simulink library "ADV_IP_MASTER"  (Simulink 8.6)
settings: Solver=VariableStepAuto  StartTime=0.0  StopTime=10.0  RelTol=1e-3
libraries: cdsEpicsOut x45, cdsFiltCtrl x25, cdsFilt x19, cdsEpicsIn x16, cdsTP x6, cdsMuxMatrix x4, VIS_LIB x1, cdsRampMuxMatrix x1, cdsFunctionCall x1, SIXOSEM_F_WD_AC_MASTER x1, SIXOSEM_F_STAGE_MASTER x1
(part 1 of 5)
settings Model: Creator=controls  LastModifiedBy=controls

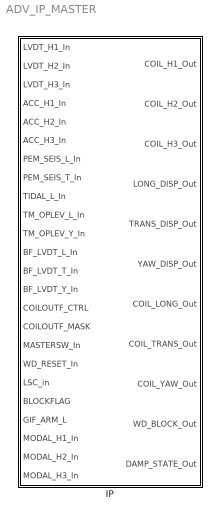
== system ADV_IP_MASTER ==
  IP : Subsystem

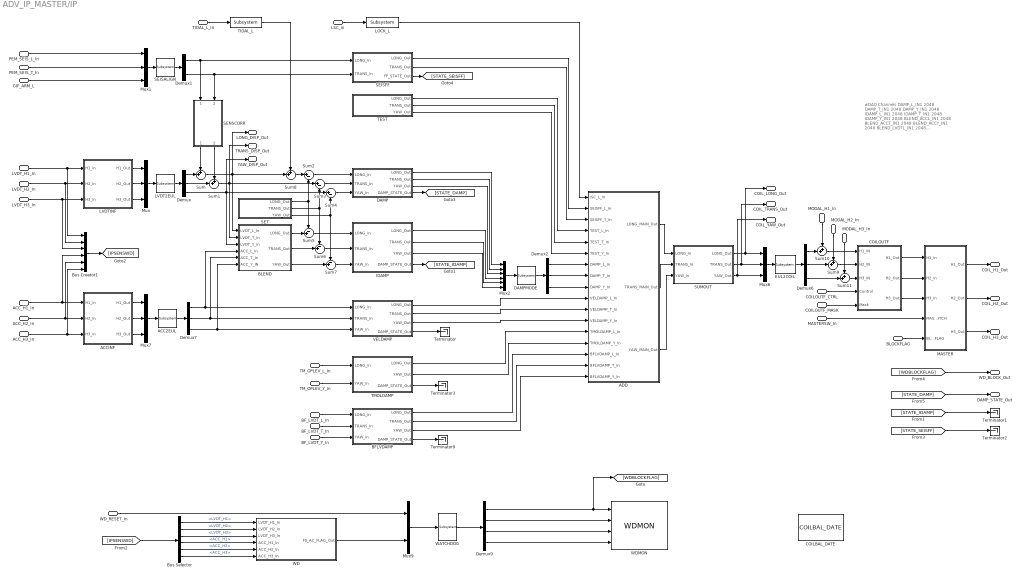
== system ADV_IP_MASTER/IP ==
  note: #DAQ Channels
      | DAMP_L_IN1 2048
      | DAMP_T_IN1 2048
      | DAMP_Y_IN1 2048
      | IDAMP_L_IN1 2048
      | IDAMP_T_IN1 2048
      | IDAMP_Y_IN1 2048
      | BLEND_ACCL_IN1 2048
      | BLEND_ACCT_IN1 2048
      | BLEND_ACCY_IN1 2048
      | BLEND_LVDTL_IN1 2048
      | BLEND_LVDTT_IN1 2048
      | BLEND_LVDTY_IN1 2048
      | DAMP_L_OUT 256
      | DAMP_T_OUT 256
      | DAMP_Y_OUT 256
      | IDAMP_L_OUT 256
      | IDAMP_T_OUT 256
      | IDAMP_Y_OUT 256
      | SEISFF_L_OUT 256
      | SEISFF_T_OUT 256
      | LOCK_L_OUT 256
      | TIDAL_L_OUT 32
  LVDT_H1_In : Inport
  LVDT_H2_In : Inport  Port=2
  LVDT_H3_In : Inport  Port=3
  ACC_H1_In : Inport  Port=4
  ACC_H2_In : Inport  Port=5
  ACC_H3_In : Inport  Port=6
  PEM_SEIS_L_In : Inport  Port=7
  PEM_SEIS_T_In : Inport  Port=8
  TIDAL_L_In : Inport  Port=9
  TM_OPLEV_L_In : Inport  Port=10
  TM_OPLEV_Y_In : Inport  Port=11
  BF_LVDT_L_In : Inport  Port=12
  BF_LVDT_T_In : Inport  Port=13
  BF_LVDT_Y_In : Inport  Port=14
  COILOUTF_CTRL : Inport  Port=15
  COILOUTF_MASK : Inport  Port=16
  MASTERSW_In : Inport  Port=17
  WD_RESET_In : Inport  Port=18
  LSC_in : Inport  Port=19
  BLOCKFLAG : Inport  Port=20
  GIF_ARM_L : Inport  Port=21
  MODAL_H1_In : Inport  Port=22
  MODAL_H2_In : Inport  Port=23
  MODAL_H3_In : Inport  Port=24
  ACC2EUL : cdsMuxMatrix/Subsystem  Tag=cdsMuxMatrix  Description=|
      | ADL=SUS_INMATRIX.adl
      | SCRIPT=generate_KisselButton.py 4 5 #CHANNEL# > #TARGET_DIR#/#FULL_PART_NAME#_KB.adl
      settings: AttributesFormatString=%<Tag>
  ACCINF : Subsystem
  ADD : Subsystem
  BFLVDAMP : Subsystem
  BLEND : Subsystem
  Bus Creator1 : BusCreator  Inputs='LVDT_H1','LVDT_H2','LVDT_H3','ACC_H1','ACC_H2','ACC_H3'
  Bus Selector : BusSelector  OutputSignals=LVDT_H1,LVDT_H2,LVDT_H3,ACC_H1,ACC_H2,ACC_H3
  COILBAL_DATE : VIS_LIB/COILBAL_DATE
  COILOUTF : Subsystem
  DAMP : Subsystem
  DAMPMODE : cdsRampMuxMatrix/Subsystem  Tag=cdsRampMuxMatrix
      settings: AttributesFormatString=%<Tag>
  Demux{,2,6..7} (4 alike) : Demux  Outputs=3
  Demux1 : Demux  Outputs=2
  Demux9 : Demux
  EUL2COIL : cdsMuxMatrix/Subsystem  Tag=cdsMuxMatrix  Description=|
      | ADL=SUS_INMATRIX.adl
      | SCRIPT=generate_KisselButton.py 4 5 #CHANNEL# > #TARGET_DIR#/#FULL_PART_NAME#_KB.adl
      settings: AttributesFormatString=%<Tag>
  IDAMP : Subsystem
  LOCK_L : cdsFilt/Subsystem  Tag=cdsFilt  Description=|
      | Purpose:                                                                                                                                                                                                                                  
      | Standard CDS IIR filter module.                                                                                                                                                                                                           
      |                                                                                                                                                                                                                                           
      | Operation:                                                                                                                                                                                                                                
      | Consists of 10 second order section IIR filters, plus a ramped gain stage. In FE code, also provides pre-defined test points and excitation channel inputs. The filter coefficients are defined in the LIGO system using the 'foton' tool.
      |                                                                                                                                                                                                                                           
      | Usage:                                                                                                                                                                                                                                    
      | Name the part with the desired filter module name.
      settings: AttributesFormatString=%<Tag>
  LVDT2EUL : cdsMuxMatrix/Subsystem  Tag=cdsMuxMatrix  Description=|
      | ADL=SUS_INMATRIX.adl
      | SCRIPT=generate_KisselButton.py 4 5 #CHANNEL# > #TARGET_DIR#/#FULL_PART_NAME#_KB.adl
      settings: AttributesFormatString=%<Tag>
  LVDTINF : Subsystem
  MASTER : Subsystem
  Mux{,1,6..7} (4 alike) : Mux  Inputs=3
  Mux2 : Mux  Inputs=6
  Mux9 : Mux  Inputs=2
  SEISALIGN : cdsMuxMatrix/Subsystem  Tag=cdsMuxMatrix  Description=|
      | ADL=SUS_INMATRIX.adl
      | SCRIPT=generate_KisselButton.py 4 5 #CHANNEL# > #TARGET_DIR#/#FULL_PART_NAME#_KB.adl
      settings: AttributesFormatString=%<Tag>
  SEISFF : Subsystem
  SENSCORR : Subsystem
  SET : Subsystem
  SUMOUT : Subsystem
  Sum{,1,8..11} (6 alike) : Sum  Inputs=++|
  Sum2 : Sum  Inputs=|+-
  Sum3 : Sum  Inputs=|+-
  Sum4 : Sum  Inputs=|+-
  Sum5 : Sum  Inputs=-+|
  Sum6 : Sum  Inputs=-+|
  Sum7 : Sum  Inputs=-+|
  TEST : Subsystem
  TIDAL_L : cdsFilt/Subsystem  Tag=cdsFilt  Description=|
      | Purpose:                                                                                                                                                                                                                                  
      | Standard CDS IIR filter module.                                                                                                                                                                                                           
      |                                                                                                                                                                                                                                           
      | Operation:                                                                                                                                                                                                                                
      | Consists of 10 second order section IIR filters, plus a ramped gain stage. In FE code, also provides pre-defined test points and excitation channel inputs. The filter coefficients are defined in the LIGO system using the 'foton' tool.
      |                                                                                                                                                                                                                                           
      | Usage:                                                                                                                                                                                                                                    
      | Name the part with the desired filter module name.
      settings: AttributesFormatString=%<Tag>
  TMOLDAMP : Subsystem
  Terminator{,1..3,9} (5 alike) : Terminator
  VELDAMP : Subsystem
  WATCHDOG : cdsFunctionCall/Subsystem  Tag=cdsFunctionCall  Description=inline OSEMWATCHDOG /opt/rtcds/userapps/release/vis/common/src/WATCHDOG.c
      settings: AttributesFormatString=%<Tag>\n%<Description>
  WD : Subsystem
  WDMON : SIXOSEM_F_STAGE_MASTER/SIXOSEM_F_STAGE_MASTER/WDMON
  COIL_H1_Out : Outport
  COIL_H2_Out : Outport  Port=2
  COIL_H3_Out : Outport  Port=3
  LONG_DISP_Out : Outport  Port=4
  TRANS_DISP_Out : Outport  Port=5
  YAW_DISP_Out : Outport  Port=6
  COIL_LONG_Out : Outport  Port=7
  COIL_TRANS_Out : Outport  Port=8
  COIL_YAW_Out : Outport  Port=9
  WD_BLOCK_Out : Outport  Port=10
  DAMP_STATE_Out : Outport  Port=11
  wires:
  MODAL_H3_In/1 -> Sum11/1
  MODAL_H2_In/1 -> Sum9/1
  Demux6/3 -> Sum11/2
  Sum11/1 -> COILOUTF/3(H3_IN)
  Sum9/1 -> COILOUTF/2(H2_IN)
  Demux6/2 -> Sum9/2
  Sum10/1 -> COILOUTF/1(H1_IN)
  Demux6/1 -> Sum10/2
  MODAL_H1_In/1 -> Sum10/1
  [STATE_DAMP] -> DAMP_STATE_Out/1
  [WDBLOCKFLAG] -> WD_BLOCK_Out/1
  COILOUTF_MASK/1 -> COILOUTF/5(Mask)
  COILOUTF_CTRL/1 -> COILOUTF/4(Control)
  TEST/3(YAW_Out) -> ADD/6(TEST_Y_In)
  TEST/2(TRANS_Out) -> ADD/5(TEST_T_In)
  TEST/1(LONG_Out) -> ADD/4(TEST_L_In)
  BLEND/3(YAW_Out) -> Sum7/2
  BLEND/2(TRANS_Out) -> Sum6/2
  BLOCKFLAG/1 -> MASTER/5(BLOCKFLAG)
  Bus Creator1/1 -> [IPSENSWD]
  ACC_H3_In/1 -> ACCINF/3(H3_In), Bus Creator1/6
  ACC_H2_In/1 -> ACCINF/2(H2_In), Bus Creator1/5
  ACC_H1_In/1 -> ACCINF/1(H1_In), Bus Creator1/4
  LVDT_H3_In/1 -> LVDTINF/3(H3_In), Bus Creator1/3
  LVDT_H2_In/1 -> LVDTINF/2(H2_In), Bus Creator1/2
  LVDT_H1_In/1 -> LVDTINF/1(H1_In), Bus Creator1/1
  WATCHDOG/1 -> Demux9/1
  Mux9/1 -> WATCHDOG/1
  Demux9/4 -> WDMON/4
  Demux9/3 -> WDMON/3
  Demux9/2 -> WDMON/2
  Demux9/1 -> WDMON/1, [WDBLOCKFLAG]
  Bus Selector/5 -> WD/5(ACC_H2_In)  "<ACC_H2>"
  Bus Selector/6 -> WD/6(ACC_H3_In)  "<ACC_H3>"
  Bus Selector/4 -> WD/4(ACC_H1_In)  "<ACC_H1>"
  Bus Selector/3 -> WD/3(LVDT_H3_In)  "<LVDT_H3>"
  Bus Selector/2 -> WD/2(LVDT_H2_In)  "<LVDT_H2>"
  Bus Selector/1 -> WD/1(LVDT_H1_In)  "<LVDT_H1>"
  [IPSENSWD] -> Bus Selector/1
  WD/1(F0_AC_FLAG_Out) -> Mux9/2
  WD_RESET_In/1 -> Mux9/1
  MASTERSW_In/1 -> MASTER/4(MASTERSWITCH)
  COILOUTF/3(H3_Out) -> MASTER/3(H3_In)
  COILOUTF/2(H2_Out) -> MASTER/2(H2_In)
  COILOUTF/1(H1_Out) -> MASTER/1(H1_In)
  MASTER/3(H3_Out) -> COIL_H3_Out/1
  MASTER/2(H2_Out) -> COIL_H2_Out/1
  MASTER/1(H1_Out) -> COIL_H1_Out/1
  EUL2COIL/1 -> Demux6/1
  Mux6/1 -> EUL2COIL/1
  Demux7/3 -> BLEND/6(ACC_Y_IN), VELDAMP/3(YAW_In)
  Demux7/2 -> BLEND/5(ACC_T_In), VELDAMP/2(TRANS_In)
  Demux7/1 -> BLEND/4(ACC_L_In), VELDAMP/1(LONG_In)
  Demux/3 -> Sum4/1, BLEND/3(LVDT_Y_In), YAW_DISP_Out/1
  Sum1/1 -> Sum3/1, BLEND/2(LVDT_T_In), TRANS_DISP_Out/1
  Sum/1 -> Sum8/2, LONG_DISP_Out/1, BLEND/1(LVDT_L_In)
  ACC2EUL/1 -> Demux7/1
  ACCINF/2(H2_Out) -> Mux7/2
  ACCINF/3(H3_Out) -> Mux7/3
  ACCINF/1(H1_Out) -> Mux7/1
  Mux7/1 -> ACC2EUL/1
  LVDT2EUL/1 -> Demux/1
  Mux/1 -> LVDT2EUL/1
  LVDTINF/3(H3_Out) -> Mux/3
  LVDTINF/2(H2_Out) -> Mux/2
  LVDTINF/1(H1_Out) -> Mux/1
  VELDAMP/1(LONG_Out) -> ADD/10(VELDAMP_L_In)
  VELDAMP/2(TRANS_Out) -> ADD/11(VELDAMP_T_In)
  VELDAMP/3(YAW_Out) -> ADD/12(VELDAMP_Y_In)
  VELDAMP/4(DAMP_STATE_Out) -> Terminator/1
  LSC_in/1 -> LOCK_L/1
  BLEND/1(LONG_Out) -> Sum5/2
  DAMP/4(DAMP_STATE_Out) -> [STATE_DAMP]
  IDAMP/4(DAMP_STATE_Out) -> [STATE_IDAMP]
  [STATE_IDAMP] -> Terminator1/1
  Demux/1 -> Sum/2
  SENSCORR/1(SC_L_Out) -> Sum/1
  Demux/2 -> Sum1/2
  SENSCORR/2(SC_T_Out) -> Sum1/1
  SEISFF/3(FF_STATE_Out) -> [STATE_SEISFF]
  SEISFF/2(TRANS_Out) -> ADD/3(SEISFF_T_In)
  SEISFF/1(LONG_Out) -> ADD/2(SEISFF_L_In)
  [STATE_SEISFF] -> Terminator2/1
  SUMOUT/3(YAW_Out) -> COIL_YAW_Out/1, Mux6/3
  SUMOUT/1(LONG_Out) -> COIL_LONG_Out/1, Mux6/1
  SUMOUT/2(TRANS_Out) -> COIL_TRANS_Out/1, Mux6/2
  ADD/2(TRANS_MAIN_Out) -> SUMOUT/2(TRANS_In)
  ADD/1(LONG_MAIN_Out) -> SUMOUT/1(LONG_In)
  ADD/3(YAW_MAIN_Out) -> SUMOUT/3(YAW_In)
  PEM_SEIS_T_In/1 -> Mux1/2
  PEM_SEIS_L_In/1 -> Mux1/1
  Mux1/1 -> SEISALIGN/1
  SEISALIGN/1 -> Demux1/1
  Demux1/2 -> SENSCORR/2(SEIS_T_In), SEISFF/2(TRANS_In)
  Demux1/1 -> SENSCORR/1(SEIS_L_In), SEISFF/1(LONG_In)
  Sum2/1 -> DAMP/1(LONG_In)
  Sum3/1 -> DAMP/2(TRANS_In)
  Sum4/1 -> DAMP/3(YAW_In)
  SET/1(LONG_Out) -> Sum5/1, Sum2/2
  SET/2(TRANS_Out) -> Sum3/2, Sum6/1
  SET/3(YAW_Out) -> Sum7/1, Sum4/2
  Sum7/1 -> IDAMP/3(YAW_In)
  Sum6/1 -> IDAMP/2(TRANS_In)
  Sum5/1 -> IDAMP/1(LONG_In)
  Mux2/1 -> DAMPMODE/1
  DAMPMODE/1 -> Demux2/1
  DAMP/3(YAW_Out) -> Mux2/3
  DAMP/2(TRANS_Out) -> Mux2/2
  DAMP/1(LONG_Out) -> Mux2/1
  IDAMP/3(YAW_Out) -> Mux2/6
  IDAMP/2(TRANS_Out) -> Mux2/5
  IDAMP/1(LONG_Out) -> Mux2/4
  Demux2/1 -> ADD/7(DAMP_L_In)
  Demux2/2 -> ADD/8(DAMP_T_In)
  Demux2/3 -> ADD/9(DAMP_Y_In)
  LOCK_L/1 -> ADD/1(ISC_L_In)
  TMOLDAMP/3(DAMP_STATE_Out) -> Terminator3/1
  TM_OPLEV_L_In/1 -> TMOLDAMP/1(LONG_In)
  TM_OPLEV_Y_In/1 -> TMOLDAMP/2(YAW_In)
  BFLVDAMP/4(DAMP_STATE_Out) -> Terminator9/1
  TMOLDAMP/1(LONG_Out) -> ADD/13(TMOLDAMP_L_In)
  TMOLDAMP/2(YAW_Out) -> ADD/14(TMOLDAMP_Y_In)
  BFLVDAMP/3(YAW_Out) -> ADD/17(BFLVDAMP_Y_In)
  BFLVDAMP/2(TRANS_Out) -> ADD/16(BFLVDAMP_T_In)
  BFLVDAMP/1(LONG_Out) -> ADD/15(BFLVDAMP_L_In)
  BF_LVDT_T_In/1 -> BFLVDAMP/2(TRANS_In)
  BF_LVDT_L_In/1 -> BFLVDAMP/1(LONG_In)
  BF_LVDT_Y_In/1 -> BFLVDAMP/3(YAW_In)
  GIF_ARM_L/1 -> Mux1/3
  Sum8/1 -> Sum2/1
  TIDAL_L/1 -> Sum8/1
  TIDAL_L_In/1 -> TIDAL_L/1

== system ADV_IP_MASTER/IP/ACCINF ==
  H1_In : Inport
  H2_In : Inport  Port=2
  H3_In : Inport  Port=3
  H1 : cdsFilt/Subsystem  Tag=cdsFilt  Description=|
      | Purpose:                                                                                                                                                                                                                                  
      | Standard CDS IIR filter module.                                                                                                                                                                                                           
      |                                                                                                                                                                                                                                           
      | Operation:                                                                                                                                                                                                                                
      | Consists of 10 second order section IIR filters, plus a ramped gain stage. In FE code, also provides pre-defined test points and excitation channel inputs. The filter coefficients are defined in the LIGO system using the 'foton' tool.
      |                                                                                                                                                                                                                                           
      | Usage:                                                                                                                                                                                                                                    
      | Name the part with the desired filter module name.
      settings: AttributesFormatString=%<Tag>
  H2 : cdsFilt/Subsystem  Tag=cdsFilt  Description=|
      | Purpose:                                                                                                                                                                                                                                  
      | Standard CDS IIR filter module.                                                                                                                                                                                                           
      |                                                                                                                                                                                                                                           
      | Operation:                                                                                                                                                                                                                                
      | Consists of 10 second order section IIR filters, plus a ramped gain stage. In FE code, also provides pre-defined test points and excitation channel inputs. The filter coefficients are defined in the LIGO system using the 'foton' tool.
      |                                                                                                                                                                                                                                           
      | Usage:                                                                                                                                                                                                                                    
      | Name the part with the desired filter module name.
      settings: AttributesFormatString=%<Tag>
  H3 : cdsFilt/Subsystem  Tag=cdsFilt  Description=|
      | Purpose:                                                                                                                                                                                                                                  
      | Standard CDS IIR filter module.                                                                                                                                                                                                           
      |                                                                                                                                                                                                                                           
      | Operation:                                                                                                                                                                                                                                
      | Consists of 10 second order section IIR filters, plus a ramped gain stage. In FE code, also provides pre-defined test points and excitation channel inputs. The filter coefficients are defined in the LIGO system using the 'foton' tool.
      |                                                                                                                                                                                                                                           
      | Usage:                                                                                                                                                                                                                                    
      | Name the part with the desired filter module name.
      settings: AttributesFormatString=%<Tag>
  H1_Out : Outport
  H2_Out : Outport  Port=2
  H3_Out : Outport  Port=3
  wires:
  H3/1 -> H3_Out/1
  H3_In/1 -> H3/1
  H2/1 -> H2_Out/1
  H2_In/1 -> H2/1
  H1/1 -> H1_Out/1
  H1_In/1 -> H1/1

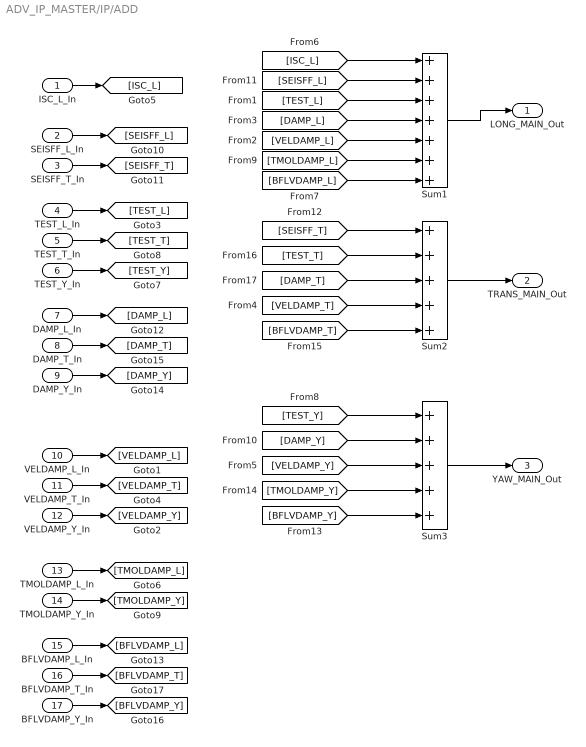
== system ADV_IP_MASTER/IP/ADD ==
  ISC_L_In : Inport
  SEISFF_L_In : Inport  Port=2
  SEISFF_T_In : Inport  Port=3
  TEST_L_In : Inport  Port=4
  TEST_T_In : Inport  Port=5
  TEST_Y_In : Inport  Port=6
  DAMP_L_In : Inport  Port=7
  DAMP_T_In : Inport  Port=8
  DAMP_Y_In : Inport  Port=9
  VELDAMP_L_In : Inport  Port=10
  VELDAMP_T_In : Inport  Port=11
  VELDAMP_Y_In : Inport  Port=12
  TMOLDAMP_L_In : Inport  Port=13
  TMOLDAMP_Y_In : Inport  Port=14
  BFLVDAMP_L_In : Inport  Port=15
  BFLVDAMP_T_In : Inport  Port=16
  BFLVDAMP_Y_In : Inport  Port=17
  Sum1 : Sum  Inputs=+++++++
  Sum2 : Sum  Inputs=+++++
  Sum3 : Sum  Inputs=+++++
  LONG_MAIN_Out : Outport
  TRANS_MAIN_Out : Outport  Port=2
  YAW_MAIN_Out : Outport  Port=3
  wires:
  [DAMP_Y] -> Sum3/2
  [TEST_Y] -> Sum3/1
  Sum3/1 -> YAW_MAIN_Out/1
  Sum2/1 -> TRANS_MAIN_Out/1
  DAMP_Y_In/1 -> [DAMP_Y]
  DAMP_T_In/1 -> [DAMP_T]
  DAMP_L_In/1 -> [DAMP_L]
  TEST_Y_In/1 -> [TEST_Y]
  TEST_T_In/1 -> [TEST_T]
  TEST_L_In/1 -> [TEST_L]
  Sum1/1 -> LONG_MAIN_Out/1
  VELDAMP_Y_In/1 -> [VELDAMP_Y]
  VELDAMP_T_In/1 -> [VELDAMP_T]
  VELDAMP_L_In/1 -> [VELDAMP_L]
  [VELDAMP_Y] -> Sum3/3
  SEISFF_T_In/1 -> [SEISFF_T]
  SEISFF_L_In/1 -> [SEISFF_L]
  [SEISFF_T] -> Sum2/1
  [TEST_T] -> Sum2/2
  [DAMP_T] -> Sum2/3
  [VELDAMP_T] -> Sum2/4
  ISC_L_In/1 -> [ISC_L]
  [TEST_L] -> Sum1/3
  [SEISFF_L] -> Sum1/2
  [VELDAMP_L] -> Sum1/5
  [DAMP_L] -> Sum1/4
  [ISC_L] -> Sum1/1
  TMOLDAMP_Y_In/1 -> [TMOLDAMP_Y]
  TMOLDAMP_L_In/1 -> [TMOLDAMP_L]
  BFLVDAMP_Y_In/1 -> [BFLVDAMP_Y]
  BFLVDAMP_T_In/1 -> [BFLVDAMP_T]
  BFLVDAMP_L_In/1 -> [BFLVDAMP_L]
  [TMOLDAMP_L] -> Sum1/6
  [BFLVDAMP_L] -> Sum1/7
  [BFLVDAMP_Y] -> Sum3/5
  [TMOLDAMP_Y] -> Sum3/4
  [BFLVDAMP_T] -> Sum2/5

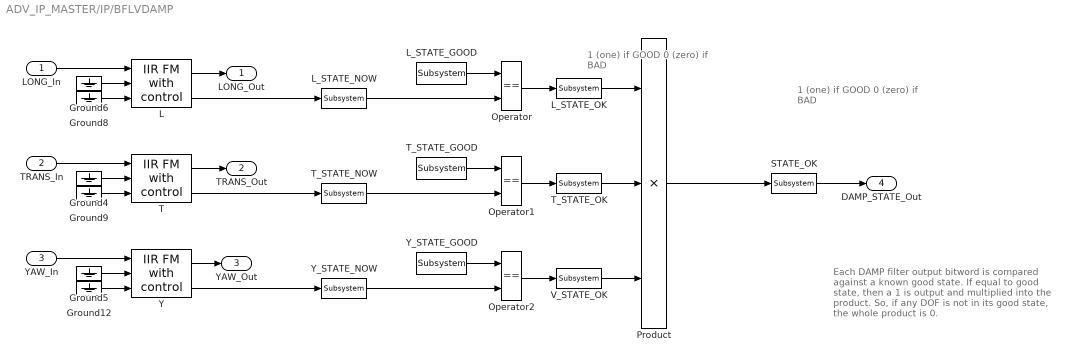
== system ADV_IP_MASTER/IP/BFLVDAMP ==
  note: 1 (one) if GOOD
      | 0 (zero) if BAD
  note: 1 (one) if GOOD
      | 0 (zero) if BAD
  note: Each DAMP filter output bitword is
      | compared against a known good state.
      | If equal to good state, then a 1 is output
      | and multiplied into the product. So, if any DOF
      | is not in its good state, the whole product is 0.
  LONG_In : Inport
  TRANS_In : Inport  Port=2
  YAW_In : Inport  Port=3
  Ground{4..6,8..9,12} (6 alike) : Ground
  L : cdsFiltCtrl/IIR FM with control  Tag=cdsFiltCtrl  Description=|
      | cdsFiltCntrl is the standard IIR filter module (exactly the same as cdsFilt) but with added control data output 'Ctrl'. Filter module digital signal output appears on the first output, which is called 'Val'. 'Ctrl' output has a bit pattern encoding the state of filter's on/off switches (FM1 through FM10). The bit values are:
      |                                                                                                                                                                                                                                                                                                                                       
      | module 	hex	dec                                                                                                                                                                                                                                                                                                                       
      | -----------------------                                                                                                                                                                                                                                                                                                               
      | FM1	0x20                    32                                                                                                                                                                                                                                                                                                        
      | FM2	0x80                     128                                                                                                                                                                                                                                                                                                      
      | FM3	0x200                   512                                                                                                                                                                                                                                                                                                       
      | FM4	0x800                   2048                                                                                                                                                                                                                                                                                                      
      | FM5	0x2000                 8192                                                                                                                                                                                                                                                                                                       
      | FM6	0x8000                 32768                                                                                                                                                                                                                                                                                                      
      | FM7	0x20000                131072                                                                                                                                                                                                                                                                                                     
      | FM8	0x80000                 524288                                                                                                                                                                                                                                                                                                    
      | FM9	0x200000               2097152                                                                                                                                                                                                                                                                                                    
      | FM10	0x800000               8388608                                                                                                                                                                                                                                                                                                   
      |                                                                                                                                                                                                                                                                                                                                       
      | This bit data can be used to drive some other switches or it can be output using a binary I/O module.
      settings: AttributesFormatString=%<Tag>
  L_STATE_GOOD : cdsEpicsIn/Subsystem  Tag=cdsEpicsIn  Description=|
      | Purpose:                                                                              
      | Create an EPICS input channel connection to the FE realtime controls.                 
      |                                                                                       
      | Operation:                                                                            
      | Outputs value from an EPICS ai record. Value is floating point with a precision of 3..
      |                                                                                       
      | Usage:                                                                                
      | Name the part with the desired EPICS channel name.
      settings: AttributesFormatString=%<Tag>
  L_STATE_NOW : cdsEpicsOut/Subsystem  Tag=cdsEpicsOutput  Description=|
      | Purpose:                                          
      | Output a FE signal to an EPICS channel.           
      |                                                   
      | Operation:                                        
      | Takes input value and passes it to EPICS record.  
      |                                                   
      | Usage:                                            
      | Name the part with the desired EPICS rrecord name.
      settings: AttributesFormatString=%<Tag>
  L_STATE_OK : cdsEpicsOut/Subsystem  Tag=cdsEpicsOutput  Description=|
      | Purpose:                                          
      | Output a FE signal to an EPICS channel.           
      |                                                   
      | Operation:                                        
      | Takes input value and passes it to EPICS record.  
      |                                                   
      | Usage:                                            
      | Name the part with the desired EPICS rrecord name.
      settings: AttributesFormatString=%<Tag>
  Operator : RelationalOperator  Operator===  OutDataTypeStr=boolean
  Operator1 : RelationalOperator  Operator===  OutDataTypeStr=boolean
  Operator2 : RelationalOperator  Operator===  OutDataTypeStr=boolean
  Product : Product  Inputs=3  RndMeth=Zero
  STATE_OK : cdsEpicsOut/Subsystem  Tag=cdsEpicsOutput  Description=|
      | Purpose:                                          
      | Output a FE signal to an EPICS channel.           
      |                                                   
      | Operation:                                        
      | Takes input value and passes it to EPICS record.  
      |                                                   
      | Usage:                                            
      | Name the part with the desired EPICS rrecord name.
      settings: AttributesFormatString=%<Tag>
  T : cdsFiltCtrl/IIR FM with control  Tag=cdsFiltCtrl  Description=|
      | cdsFiltCntrl is the standard IIR filter module (exactly the same as cdsFilt) but with added control data output 'Ctrl'. Filter module digital signal output appears on the first output, which is called 'Val'. 'Ctrl' output has a bit pattern encoding the state of filter's on/off switches (FM1 through FM10). The bit values are:
      |                                                                                                                                                                                                                                                                                                                                       
      | module 	hex	dec                                                                                                                                                                                                                                                                                                                       
      | -----------------------                                                                                                                                                                                                                                                                                                               
      | FM1	0x20                    32                                                                                                                                                                                                                                                                                                        
      | FM2	0x80                     128                                                                                                                                                                                                                                                                                                      
      | FM3	0x200                   512                                                                                                                                                                                                                                                                                                       
      | FM4	0x800                   2048                                                                                                                                                                                                                                                                                                      
      | FM5	0x2000                 8192                                                                                                                                                                                                                                                                                                       
      | FM6	0x8000                 32768                                                                                                                                                                                                                                                                                                      
      | FM7	0x20000                131072                                                                                                                                                                                                                                                                                                     
      | FM8	0x80000                 524288                                                                                                                                                                                                                                                                                                    
      | FM9	0x200000               2097152                                                                                                                                                                                                                                                                                                    
      | FM10	0x800000               8388608                                                                                                                                                                                                                                                                                                   
      |                                                                                                                                                                                                                                                                                                                                       
      | This bit data can be used to drive some other switches or it can be output using a binary I/O module.
      settings: AttributesFormatString=%<Tag>
  T_STATE_GOOD : cdsEpicsIn/Subsystem  Tag=cdsEpicsIn  Description=|
      | Purpose:                                                                              
      | Create an EPICS input channel connection to the FE realtime controls.                 
      |                                                                                       
      | Operation:                                                                            
      | Outputs value from an EPICS ai record. Value is floating point with a precision of 3..
      |                                                                                       
      | Usage:                                                                                
      | Name the part with the desired EPICS channel name.
      settings: AttributesFormatString=%<Tag>
  T_STATE_NOW : cdsEpicsOut/Subsystem  Tag=cdsEpicsOutput  Description=|
      | Purpose:                                          
      | Output a FE signal to an EPICS channel.           
      |                                                   
      | Operation:                                        
      | Takes input value and passes it to EPICS record.  
      |                                                   
      | Usage:                                            
      | Name the part with the desired EPICS rrecord name.
      settings: AttributesFormatString=%<Tag>
  T_STATE_OK : cdsEpicsOut/Subsystem  Tag=cdsEpicsOutput  Description=|
      | Purpose:                                          
      | Output a FE signal to an EPICS channel.           
      |                                                   
      | Operation:                                        
      | Takes input value and passes it to EPICS record.  
      |                                                   
      | Usage:                                            
      | Name the part with the desired EPICS rrecord name.
      settings: AttributesFormatString=%<Tag>
  V_STATE_OK : cdsEpicsOut/Subsystem  Tag=cdsEpicsOutput  Description=|
      | Purpose:                                          
      | Output a FE signal to an EPICS channel.           
      |                                                   
      | Operation:                                        
      | Takes input value and passes it to EPICS record.  
      |                                                   
      | Usage:                                            
      | Name the part with the desired EPICS rrecord name.
      settings: AttributesFormatString=%<Tag>
  Y : cdsFiltCtrl/IIR FM with control  Tag=cdsFiltCtrl  Description=|
      | cdsFiltCntrl is the standard IIR filter module (exactly the same as cdsFilt) but with added control data output 'Ctrl'. Filter module digital signal output appears on the first output, which is called 'Val'. 'Ctrl' output has a bit pattern encoding the state of filter's on/off switches (FM1 through FM10). The bit values are:
      |                                                                                                                                                                                                                                                                                                                                       
      | module 	hex	dec                                                                                                                                                                                                                                                                                                                       
      | -----------------------                                                                                                                                                                                                                                                                                                               
      | FM1	0x20                    32                                                                                                                                                                                                                                                                                                        
      | FM2	0x80                     128                                                                                                                                                                                                                                                                                                      
      | FM3	0x200                   512                                                                                                                                                                                                                                                                                                       
      | FM4	0x800                   2048                                                                                                                                                                                                                                                                                                      
      | FM5	0x2000                 8192                                                                                                                                                                                                                                                                                                       
      | FM6	0x8000                 32768                                                                                                                                                                                                                                                                                                      
      | FM7	0x20000                131072                                                                                                                                                                                                                                                                                                     
      | FM8	0x80000                 524288                                                                                                                                                                                                                                                                                                    
      | FM9	0x200000               2097152                                                                                                                                                                                                                                                                                                    
      | FM10	0x800000               8388608                                                                                                                                                                                                                                                                                                   
      |                                                                                                                                                                                                                                                                                                                                       
      | This bit data can be used to drive some other switches or it can be output using a binary I/O module.
      settings: AttributesFormatString=%<Tag>
  Y_STATE_GOOD : cdsEpicsIn/Subsystem  Tag=cdsEpicsIn  Description=|
      | Purpose:                                                                              
      | Create an EPICS input channel connection to the FE realtime controls.                 
      |                                                                                       
      | Operation:                                                                            
      | Outputs value from an EPICS ai record. Value is floating point with a precision of 3..
      |                                                                                       
      | Usage:                                                                                
      | Name the part with the desired EPICS channel name.
      settings: AttributesFormatString=%<Tag>
  Y_STATE_NOW : cdsEpicsOut/Subsystem  Tag=cdsEpicsOutput  Description=|
      | Purpose:                                          
      | Output a FE signal to an EPICS channel.           
      |                                                   
      | Operation:                                        
      | Takes input value and passes it to EPICS record.  
      |                                                   
      | Usage:                                            
      | Name the part with the desired EPICS rrecord name.
      settings: AttributesFormatString=%<Tag>
  LONG_Out : Outport
  TRANS_Out : Outport  Port=2
  YAW_Out : Outport  Port=3
  DAMP_STATE_Out : Outport  Port=4
  wires:
  Ground12/1 -> Y/3
  Ground9/1 -> T/3
  Ground8/1 -> L/3
  STATE_OK/1 -> DAMP_STATE_Out/1
  Y_STATE_NOW/1 -> Operator2/2
  T_STATE_NOW/1 -> Operator1/2
  L_STATE_NOW/1 -> Operator/2
  V_STATE_OK/1 -> Product/3
  T_STATE_OK/1 -> Product/2
  L_STATE_OK/1 -> Product/1
  Operator2/1 -> V_STATE_OK/1
  Operator1/1 -> T_STATE_OK/1
  Operator/1 -> L_STATE_OK/1
  Product/1 -> STATE_OK/1
  Y/2 -> Y_STATE_NOW/1
  Y_STATE_GOOD/1 -> Operator2/1
  T/2 -> T_STATE_NOW/1
  T_STATE_GOOD/1 -> Operator1/1
  L/2 -> L_STATE_NOW/1
  L_STATE_GOOD/1 -> Operator/1
  TRANS_In/1 -> T/1
  YAW_In/1 -> Y/1
  T/1 -> TRANS_Out/1
  Y/1 -> YAW_Out/1
  L/1 -> LONG_Out/1
  LONG_In/1 -> L/1
  Ground5/1 -> Y/2
  Ground4/1 -> T/2
  Ground6/1 -> L/2
